simulink model "model_2"  (R2018b)
settings: Solver=FixedStepAuto  StartTime=0.0  StopTime=100  FixedStep=0.0001  MinStep=0.00001  RelTol=1e-5  AbsTol=1e-5
values from neighbouring files (symbols this model uses):
  m = 1    [Drive.m]    (also in on.m)
  N = 1 / T_f    (= 12.8205128205)    [regler.m]
undefined symbols (not defined in the file or in its folder): X, Y, Z
libraries: sm_lib x72, nesl_utility x28, simulink x5, Contact_Forces_Lib x4, simulink_extras x3, vrlib x1
(part 3 of 3)

== system model_2/World/Tracksystem/SensorN6 ==
  Constant : Constant  Value=linePath
  Constant1 : Constant  Value=thickness
  Gain : Gain  Gain=-1
  Gain1 : Gain  Gain=-1
  MATLAB Function2 : MATLAB Function  TreatAsAtomicUnit=on
  PS-Simulink Converter : nesl_utility/PS-Simulink Converter  PhysicalDomain=network_engine_domain  SubClassName=ps_output  LeftPortType=input  RightPortType=output  PseudoPeriodic=off  Frequencies=[]  Unit=1  AffineConversion=off
  PS-Simulink Converter1 : nesl_utility/PS-Simulink Converter  PhysicalDomain=network_engine_domain  SubClassName=ps_output  LeftPortType=input  RightPortType=output  PseudoPeriodic=off  Frequencies=[]  Unit=1  AffineConversion=off
  Scope : Scope  NumInputPorts=2
  Transform Sensor : sm_lib/Frames and Transforms/Transform Sensor  MeasurementFrame=World  SenseAngle=off  SenseAxis=off  SenseAngle1=off  SenseAngle2=off  SenseAngle3=off  SenseQ=off  SenseR=off  SenseOmegaX=off  SenseOmegaY=off  SenseOmegaZ=off  SenseOmega1=off  SenseOmega2=off  SenseOmega3=off  SenseQDot=off  SenseRDot=off  SenseAlphaX=off  SenseAlphaY=off  SenseAlphaZ=off  SenseAlpha1=off  SenseAlpha2=off  SenseAlpha3=off  SenseQDDot=off  SenseRDDot=off  SenseX=on  SenseY=on  SenseZ=off  SenseRad=off  SenseAzim=off  SenseDist=off  SenseInc=off  SenseXDot=off  SenseYDot=off  SenseZDot=off  SenseRadDot=off  SenseAzimDot=off  SenseDistDot=off  SenseIncDot=off  SenseXDDot=off  SenseYDDot=off  SenseZDDot=off  SenseRadDDot=off  SenseAzimDDot=off  SenseDistDDot=off  SenseIncDDot=off
  B : PMIOPort  Side=Left
  Active : Outport
  wires:
  Constant1/1 -> MATLAB Function2/4(thickness)
  Constant/1 -> MATLAB Function2/3(linePath)
  MATLAB Function2/1(b) -> Active/1
  PS-Simulink Converter1/1 -> Gain1/1
  PS-Simulink Converter/1 -> Gain/1
  Gain/1 -> Scope/1, MATLAB Function2/1(x)
  Gain1/1 -> Scope/2, MATLAB Function2/2(y)
  connections:
  Transform Sensor/RConn3 -- PS-Simulink Converter1/LConn1
  Transform Sensor/RConn2 -- PS-Simulink Converter/LConn1
  Transform Sensor/LConn1 -- B/RConn1

== system model_2/World/Tracksystem/SensorN7 ==
  Constant : Constant  Value=linePath
  Constant1 : Constant  Value=thickness
  Gain : Gain  Gain=-1
  Gain1 : Gain  Gain=-1
  MATLAB Function2 : MATLAB Function  TreatAsAtomicUnit=on
  PS-Simulink Converter : nesl_utility/PS-Simulink Converter  PhysicalDomain=network_engine_domain  SubClassName=ps_output  LeftPortType=input  RightPortType=output  PseudoPeriodic=off  Frequencies=[]  Unit=1  AffineConversion=off
  PS-Simulink Converter1 : nesl_utility/PS-Simulink Converter  PhysicalDomain=network_engine_domain  SubClassName=ps_output  LeftPortType=input  RightPortType=output  PseudoPeriodic=off  Frequencies=[]  Unit=1  AffineConversion=off
  Scope : Scope  NumInputPorts=2
  Transform Sensor : sm_lib/Frames and Transforms/Transform Sensor  MeasurementFrame=World  SenseAngle=off  SenseAxis=off  SenseAngle1=off  SenseAngle2=off  SenseAngle3=off  SenseQ=off  SenseR=off  SenseOmegaX=off  SenseOmegaY=off  SenseOmegaZ=off  SenseOmega1=off  SenseOmega2=off  SenseOmega3=off  SenseQDot=off  SenseRDot=off  SenseAlphaX=off  SenseAlphaY=off  SenseAlphaZ=off  SenseAlpha1=off  SenseAlpha2=off  SenseAlpha3=off  SenseQDDot=off  SenseRDDot=off  SenseX=on  SenseY=on  SenseZ=off  SenseRad=off  SenseAzim=off  SenseDist=off  SenseInc=off  SenseXDot=off  SenseYDot=off  SenseZDot=off  SenseRadDot=off  SenseAzimDot=off  SenseDistDot=off  SenseIncDot=off  SenseXDDot=off  SenseYDDot=off  SenseZDDot=off  SenseRadDDot=off  SenseAzimDDot=off  SenseDistDDot=off  SenseIncDDot=off
  B : PMIOPort  Side=Left
  Active : Outport
  wires:
  Constant1/1 -> MATLAB Function2/4(thickness)
  Constant/1 -> MATLAB Function2/3(linePath)
  MATLAB Function2/1(b) -> Active/1
  PS-Simulink Converter1/1 -> Gain1/1
  PS-Simulink Converter/1 -> Gain/1
  Gain/1 -> Scope/1, MATLAB Function2/1(x)
  Gain1/1 -> Scope/2, MATLAB Function2/2(y)
  connections:
  Transform Sensor/RConn3 -- PS-Simulink Converter1/LConn1
  Transform Sensor/RConn2 -- PS-Simulink Converter/LConn1
  Transform Sensor/LConn1 -- B/RConn1

== system model_2/World/Tracksystem/SensorN8 ==
  Constant : Constant  Value=linePath
  Constant1 : Constant  Value=thickness
  Gain : Gain  Gain=-1
  Gain1 : Gain  Gain=-1
  MATLAB Function2 : MATLAB Function  TreatAsAtomicUnit=on
  PS-Simulink Converter : nesl_utility/PS-Simulink Converter  PhysicalDomain=network_engine_domain  SubClassName=ps_output  LeftPortType=input  RightPortType=output  PseudoPeriodic=off  Frequencies=[]  Unit=1  AffineConversion=off
  PS-Simulink Converter1 : nesl_utility/PS-Simulink Converter  PhysicalDomain=network_engine_domain  SubClassName=ps_output  LeftPortType=input  RightPortType=output  PseudoPeriodic=off  Frequencies=[]  Unit=1  AffineConversion=off
  Scope : Scope  NumInputPorts=2
  Transform Sensor : sm_lib/Frames and Transforms/Transform Sensor  MeasurementFrame=World  SenseAngle=off  SenseAxis=off  SenseAngle1=off  SenseAngle2=off  SenseAngle3=off  SenseQ=off  SenseR=off  SenseOmegaX=off  SenseOmegaY=off  SenseOmegaZ=off  SenseOmega1=off  SenseOmega2=off  SenseOmega3=off  SenseQDot=off  SenseRDot=off  SenseAlphaX=off  SenseAlphaY=off  SenseAlphaZ=off  SenseAlpha1=off  SenseAlpha2=off  SenseAlpha3=off  SenseQDDot=off  SenseRDDot=off  SenseX=on  SenseY=on  SenseZ=off  SenseRad=off  SenseAzim=off  SenseDist=off  SenseInc=off  SenseXDot=off  SenseYDot=off  SenseZDot=off  SenseRadDot=off  SenseAzimDot=off  SenseDistDot=off  SenseIncDot=off  SenseXDDot=off  SenseYDDot=off  SenseZDDot=off  SenseRadDDot=off  SenseAzimDDot=off  SenseDistDDot=off  SenseIncDDot=off
  B : PMIOPort  Side=Left
  Active : Outport
  wires:
  Constant1/1 -> MATLAB Function2/4(thickness)
  Constant/1 -> MATLAB Function2/3(linePath)
  MATLAB Function2/1(b) -> Active/1
  PS-Simulink Converter1/1 -> Gain1/1
  PS-Simulink Converter/1 -> Gain/1
  Gain/1 -> Scope/1, MATLAB Function2/1(x)
  Gain1/1 -> Scope/2, MATLAB Function2/2(y)
  connections:
  Transform Sensor/RConn3 -- PS-Simulink Converter1/LConn1
  Transform Sensor/RConn2 -- PS-Simulink Converter/LConn1
  Transform Sensor/LConn1 -- B/RConn1

== system model_2/World/Tracksystem/Subsystem ==
  sensorDownkord : sm_lib/Frames and Transforms/Rigid Transform  TranslationMethod=Cartesian  TranslationStandardOffset=0  TranslationLengthUnit=m  TranslationStandardAxis=-Z  TranslationCartesianOffset=[sensorRadius 0 75/1000]  TranslationROffset=0  TranslationROffsetUnits=m  TranslationZOffset=0  TranslationZOffsetUnits=m  TranslationThetaOffset=0  TranslationThetaOffsetUnits=deg  RotationMethod=None  RotationAngleUnits=deg  RotationStandardAxis=+Z  RotationAngle=45  RotationArbitraryAxis=[0 0 1]  FollAlignAxisA=+X  BaseAlignAxisA=+Y  FollAlignAxisB=+Y  BaseAlignAxisB=+Z  RotationSequenceAxes=FollowerAxes  RotationSequence=XYX  RotationSequenceAngles=[0 0 0]  RotationSequenceAnglesUnits=deg  RotationMatrix=[1 0 0; 0 1 0; 0 0 1]
  sensorDownkord8 : sm_lib/Frames and Transforms/Rigid Transform  TranslationMethod=None  TranslationStandardOffset=0  TranslationLengthUnit=m  TranslationStandardAxis=-Z  TranslationCartesianOffset=[sensorRadius 0 75/1000]  TranslationROffset=0  TranslationROffsetUnits=m  TranslationZOffset=0  TranslationZOffsetUnits=m  TranslationThetaOffset=0  TranslationThetaOffsetUnits=deg  RotationMethod=StandardAxis  RotationAngleUnits=deg  RotationStandardAxis=+Z  RotationAngle=angle  RotationArbitraryAxis=[0 0 1]  FollAlignAxisA=+X  BaseAlignAxisA=+Y  FollAlignAxisB=+Y  BaseAlignAxisB=+Z  RotationSequenceAxes=FollowerAxes  RotationSequence=XYX  RotationSequenceAngles=[0 0 0]  RotationSequenceAnglesUnits=deg  RotationMatrix=[1 0 0; 0 1 0; 0 0 1]
  B : PMIOPort  Side=Left
  F : PMIOPort  Port=2  Side=Right
  connections:
  sensorDownkord8/LConn1 -- B/RConn1
  sensorDownkord/LConn1 -- sensorDownkord8/RConn1
  sensorDownkord/RConn1 -- F/RConn1

== system model_2/World/Tracksystem/Subsystem1 ==
  sensorDownkord : sm_lib/Frames and Transforms/Rigid Transform  TranslationMethod=Cartesian  TranslationStandardOffset=0  TranslationLengthUnit=m  TranslationStandardAxis=-Z  TranslationCartesianOffset=[sensorRadius 0 75/1000]  TranslationROffset=0  TranslationROffsetUnits=m  TranslationZOffset=0  TranslationZOffsetUnits=m  TranslationThetaOffset=0  TranslationThetaOffsetUnits=deg  RotationMethod=None  RotationAngleUnits=deg  RotationStandardAxis=+Z  RotationAngle=45  RotationArbitraryAxis=[0 0 1]  FollAlignAxisA=+X  BaseAlignAxisA=+Y  FollAlignAxisB=+Y  BaseAlignAxisB=+Z  RotationSequenceAxes=FollowerAxes  RotationSequence=XYX  RotationSequenceAngles=[0 0 0]  RotationSequenceAnglesUnits=deg  RotationMatrix=[1 0 0; 0 1 0; 0 0 1]
  sensorDownkord8 : sm_lib/Frames and Transforms/Rigid Transform  TranslationMethod=None  TranslationStandardOffset=0  TranslationLengthUnit=m  TranslationStandardAxis=-Z  TranslationCartesianOffset=[sensorRadius 0 75/1000]  TranslationROffset=0  TranslationROffsetUnits=m  TranslationZOffset=0  TranslationZOffsetUnits=m  TranslationThetaOffset=0  TranslationThetaOffsetUnits=deg  RotationMethod=StandardAxis  RotationAngleUnits=deg  RotationStandardAxis=+Z  RotationAngle=angle  RotationArbitraryAxis=[0 0 1]  FollAlignAxisA=+X  BaseAlignAxisA=+Y  FollAlignAxisB=+Y  BaseAlignAxisB=+Z  RotationSequenceAxes=FollowerAxes  RotationSequence=XYX  RotationSequenceAngles=[0 0 0]  RotationSequenceAnglesUnits=deg  RotationMatrix=[1 0 0; 0 1 0; 0 0 1]
  B : PMIOPort  Side=Left
  F : PMIOPort  Port=2  Side=Right
  connections:
  sensorDownkord8/LConn1 -- B/RConn1
  sensorDownkord/LConn1 -- sensorDownkord8/RConn1
  sensorDownkord/RConn1 -- F/RConn1

== system model_2/World/Tracksystem/Subsystem2 ==
  sensorDownkord : sm_lib/Frames and Transforms/Rigid Transform  TranslationMethod=Cartesian  TranslationStandardOffset=0  TranslationLengthUnit=m  TranslationStandardAxis=-Z  TranslationCartesianOffset=[sensorRadius 0 75/1000]  TranslationROffset=0  TranslationROffsetUnits=m  TranslationZOffset=0  TranslationZOffsetUnits=m  TranslationThetaOffset=0  TranslationThetaOffsetUnits=deg  RotationMethod=None  RotationAngleUnits=deg  RotationStandardAxis=+Z  RotationAngle=45  RotationArbitraryAxis=[0 0 1]  FollAlignAxisA=+X  BaseAlignAxisA=+Y  FollAlignAxisB=+Y  BaseAlignAxisB=+Z  RotationSequenceAxes=FollowerAxes  RotationSequence=XYX  RotationSequenceAngles=[0 0 0]  RotationSequenceAnglesUnits=deg  RotationMatrix=[1 0 0; 0 1 0; 0 0 1]
  sensorDownkord8 : sm_lib/Frames and Transforms/Rigid Transform  TranslationMethod=None  TranslationStandardOffset=0  TranslationLengthUnit=m  TranslationStandardAxis=-Z  TranslationCartesianOffset=[sensorRadius 0 75/1000]  TranslationROffset=0  TranslationROffsetUnits=m  TranslationZOffset=0  TranslationZOffsetUnits=m  TranslationThetaOffset=0  TranslationThetaOffsetUnits=deg  RotationMethod=StandardAxis  RotationAngleUnits=deg  RotationStandardAxis=+Z  RotationAngle=angle  RotationArbitraryAxis=[0 0 1]  FollAlignAxisA=+X  BaseAlignAxisA=+Y  FollAlignAxisB=+Y  BaseAlignAxisB=+Z  RotationSequenceAxes=FollowerAxes  RotationSequence=XYX  RotationSequenceAngles=[0 0 0]  RotationSequenceAnglesUnits=deg  RotationMatrix=[1 0 0; 0 1 0; 0 0 1]
  B : PMIOPort  Side=Left
  F : PMIOPort  Port=2  Side=Right
  connections:
  sensorDownkord8/LConn1 -- B/RConn1
  sensorDownkord/LConn1 -- sensorDownkord8/RConn1
  sensorDownkord/RConn1 -- F/RConn1

== system model_2/World/Tracksystem/Subsystem3 ==
  sensorDownkord : sm_lib/Frames and Transforms/Rigid Transform  TranslationMethod=Cartesian  TranslationStandardOffset=0  TranslationLengthUnit=m  TranslationStandardAxis=-Z  TranslationCartesianOffset=[sensorRadius 0 75/1000]  TranslationROffset=0  TranslationROffsetUnits=m  TranslationZOffset=0  TranslationZOffsetUnits=m  TranslationThetaOffset=0  TranslationThetaOffsetUnits=deg  RotationMethod=None  RotationAngleUnits=deg  RotationStandardAxis=+Z  RotationAngle=45  RotationArbitraryAxis=[0 0 1]  FollAlignAxisA=+X  BaseAlignAxisA=+Y  FollAlignAxisB=+Y  BaseAlignAxisB=+Z  RotationSequenceAxes=FollowerAxes  RotationSequence=XYX  RotationSequenceAngles=[0 0 0]  RotationSequenceAnglesUnits=deg  RotationMatrix=[1 0 0; 0 1 0; 0 0 1]
  sensorDownkord8 : sm_lib/Frames and Transforms/Rigid Transform  TranslationMethod=None  TranslationStandardOffset=0  TranslationLengthUnit=m  TranslationStandardAxis=-Z  TranslationCartesianOffset=[sensorRadius 0 75/1000]  TranslationROffset=0  TranslationROffsetUnits=m  TranslationZOffset=0  TranslationZOffsetUnits=m  TranslationThetaOffset=0  TranslationThetaOffsetUnits=deg  RotationMethod=StandardAxis  RotationAngleUnits=deg  RotationStandardAxis=+Z  RotationAngle=angle  RotationArbitraryAxis=[0 0 1]  FollAlignAxisA=+X  BaseAlignAxisA=+Y  FollAlignAxisB=+Y  BaseAlignAxisB=+Z  RotationSequenceAxes=FollowerAxes  RotationSequence=XYX  RotationSequenceAngles=[0 0 0]  RotationSequenceAnglesUnits=deg  RotationMatrix=[1 0 0; 0 1 0; 0 0 1]
  B : PMIOPort  Side=Left
  F : PMIOPort  Port=2  Side=Right
  connections:
  sensorDownkord8/LConn1 -- B/RConn1
  sensorDownkord/LConn1 -- sensorDownkord8/RConn1
  sensorDownkord/RConn1 -- F/RConn1

== system model_2/World/Tracksystem/Subsystem5 ==
  sensorDownkord : sm_lib/Frames and Transforms/Rigid Transform  TranslationMethod=Cartesian  TranslationStandardOffset=0  TranslationLengthUnit=m  TranslationStandardAxis=-Z  TranslationCartesianOffset=[sensorRadius 0 75/1000]  TranslationROffset=0  TranslationROffsetUnits=m  TranslationZOffset=0  TranslationZOffsetUnits=m  TranslationThetaOffset=0  TranslationThetaOffsetUnits=deg  RotationMethod=None  RotationAngleUnits=deg  RotationStandardAxis=+Z  RotationAngle=45  RotationArbitraryAxis=[0 0 1]  FollAlignAxisA=+X  BaseAlignAxisA=+Y  FollAlignAxisB=+Y  BaseAlignAxisB=+Z  RotationSequenceAxes=FollowerAxes  RotationSequence=XYX  RotationSequenceAngles=[0 0 0]  RotationSequenceAnglesUnits=deg  RotationMatrix=[1 0 0; 0 1 0; 0 0 1]
  sensorDownkord8 : sm_lib/Frames and Transforms/Rigid Transform  TranslationMethod=None  TranslationStandardOffset=0  TranslationLengthUnit=m  TranslationStandardAxis=-Z  TranslationCartesianOffset=[sensorRadius 0 75/1000]  TranslationROffset=0  TranslationROffsetUnits=m  TranslationZOffset=0  TranslationZOffsetUnits=m  TranslationThetaOffset=0  TranslationThetaOffsetUnits=deg  RotationMethod=StandardAxis  RotationAngleUnits=deg  RotationStandardAxis=+Z  RotationAngle=angle  RotationArbitraryAxis=[0 0 1]  FollAlignAxisA=+X  BaseAlignAxisA=+Y  FollAlignAxisB=+Y  BaseAlignAxisB=+Z  RotationSequenceAxes=FollowerAxes  RotationSequence=XYX  RotationSequenceAngles=[0 0 0]  RotationSequenceAnglesUnits=deg  RotationMatrix=[1 0 0; 0 1 0; 0 0 1]
  B : PMIOPort  Side=Left
  F : PMIOPort  Port=2  Side=Right
  connections:
  sensorDownkord8/LConn1 -- B/RConn1
  sensorDownkord/LConn1 -- sensorDownkord8/RConn1
  sensorDownkord/RConn1 -- F/RConn1

== system model_2/World/Tracksystem/Subsystem6 ==
  sensorDownkord : sm_lib/Frames and Transforms/Rigid Transform  TranslationMethod=Cartesian  TranslationStandardOffset=0  TranslationLengthUnit=m  TranslationStandardAxis=-Z  TranslationCartesianOffset=[sensorRadius 0 75/1000]  TranslationROffset=0  TranslationROffsetUnits=m  TranslationZOffset=0  TranslationZOffsetUnits=m  TranslationThetaOffset=0  TranslationThetaOffsetUnits=deg  RotationMethod=None  RotationAngleUnits=deg  RotationStandardAxis=+Z  RotationAngle=45  RotationArbitraryAxis=[0 0 1]  FollAlignAxisA=+X  BaseAlignAxisA=+Y  FollAlignAxisB=+Y  BaseAlignAxisB=+Z  RotationSequenceAxes=FollowerAxes  RotationSequence=XYX  RotationSequenceAngles=[0 0 0]  RotationSequenceAnglesUnits=deg  RotationMatrix=[1 0 0; 0 1 0; 0 0 1]
  sensorDownkord8 : sm_lib/Frames and Transforms/Rigid Transform  TranslationMethod=None  TranslationStandardOffset=0  TranslationLengthUnit=m  TranslationStandardAxis=-Z  TranslationCartesianOffset=[sensorRadius 0 75/1000]  TranslationROffset=0  TranslationROffsetUnits=m  TranslationZOffset=0  TranslationZOffsetUnits=m  TranslationThetaOffset=0  TranslationThetaOffsetUnits=deg  RotationMethod=StandardAxis  RotationAngleUnits=deg  RotationStandardAxis=+Z  RotationAngle=angle  RotationArbitraryAxis=[0 0 1]  FollAlignAxisA=+X  BaseAlignAxisA=+Y  FollAlignAxisB=+Y  BaseAlignAxisB=+Z  RotationSequenceAxes=FollowerAxes  RotationSequence=XYX  RotationSequenceAngles=[0 0 0]  RotationSequenceAnglesUnits=deg  RotationMatrix=[1 0 0; 0 1 0; 0 0 1]
  B : PMIOPort  Side=Left
  F : PMIOPort  Port=2  Side=Right
  connections:
  sensorDownkord8/LConn1 -- B/RConn1
  sensorDownkord/LConn1 -- sensorDownkord8/RConn1
  sensorDownkord/RConn1 -- F/RConn1

== system model_2/World/Tracksystem/Subsystem7 ==
  sensorDownkord : sm_lib/Frames and Transforms/Rigid Transform  TranslationMethod=Cartesian  TranslationStandardOffset=0  TranslationLengthUnit=m  TranslationStandardAxis=-Z  TranslationCartesianOffset=[sensorRadius 0 75/1000]  TranslationROffset=0  TranslationROffsetUnits=m  TranslationZOffset=0  TranslationZOffsetUnits=m  TranslationThetaOffset=0  TranslationThetaOffsetUnits=deg  RotationMethod=None  RotationAngleUnits=deg  RotationStandardAxis=+Z  RotationAngle=45  RotationArbitraryAxis=[0 0 1]  FollAlignAxisA=+X  BaseAlignAxisA=+Y  FollAlignAxisB=+Y  BaseAlignAxisB=+Z  RotationSequenceAxes=FollowerAxes  RotationSequence=XYX  RotationSequenceAngles=[0 0 0]  RotationSequenceAnglesUnits=deg  RotationMatrix=[1 0 0; 0 1 0; 0 0 1]
  sensorDownkord8 : sm_lib/Frames and Transforms/Rigid Transform  TranslationMethod=None  TranslationStandardOffset=0  TranslationLengthUnit=m  TranslationStandardAxis=-Z  TranslationCartesianOffset=[sensorRadius 0 75/1000]  TranslationROffset=0  TranslationROffsetUnits=m  TranslationZOffset=0  TranslationZOffsetUnits=m  TranslationThetaOffset=0  TranslationThetaOffsetUnits=deg  RotationMethod=StandardAxis  RotationAngleUnits=deg  RotationStandardAxis=+Z  RotationAngle=angle  RotationArbitraryAxis=[0 0 1]  FollAlignAxisA=+X  BaseAlignAxisA=+Y  FollAlignAxisB=+Y  BaseAlignAxisB=+Z  RotationSequenceAxes=FollowerAxes  RotationSequence=XYX  RotationSequenceAngles=[0 0 0]  RotationSequenceAnglesUnits=deg  RotationMatrix=[1 0 0; 0 1 0; 0 0 1]
  B : PMIOPort  Side=Left
  F : PMIOPort  Port=2  Side=Right
  connections:
  sensorDownkord8/LConn1 -- B/RConn1
  sensorDownkord/LConn1 -- sensorDownkord8/RConn1
  sensorDownkord/RConn1 -- F/RConn1

== system model_2/World/Tracksystem/Subsystem8 ==
  sensorDownkord : sm_lib/Frames and Transforms/Rigid Transform  TranslationMethod=Cartesian  TranslationStandardOffset=0  TranslationLengthUnit=m  TranslationStandardAxis=-Z  TranslationCartesianOffset=[sensorRadius 0 75/1000]  TranslationROffset=0  TranslationROffsetUnits=m  TranslationZOffset=0  TranslationZOffsetUnits=m  TranslationThetaOffset=0  TranslationThetaOffsetUnits=deg  RotationMethod=None  RotationAngleUnits=deg  RotationStandardAxis=+Z  RotationAngle=45  RotationArbitraryAxis=[0 0 1]  FollAlignAxisA=+X  BaseAlignAxisA=+Y  FollAlignAxisB=+Y  BaseAlignAxisB=+Z  RotationSequenceAxes=FollowerAxes  RotationSequence=XYX  RotationSequenceAngles=[0 0 0]  RotationSequenceAnglesUnits=deg  RotationMatrix=[1 0 0; 0 1 0; 0 0 1]
  sensorDownkord8 : sm_lib/Frames and Transforms/Rigid Transform  TranslationMethod=None  TranslationStandardOffset=0  TranslationLengthUnit=m  TranslationStandardAxis=-Z  TranslationCartesianOffset=[sensorRadius 0 75/1000]  TranslationROffset=0  TranslationROffsetUnits=m  TranslationZOffset=0  TranslationZOffsetUnits=m  TranslationThetaOffset=0  TranslationThetaOffsetUnits=deg  RotationMethod=StandardAxis  RotationAngleUnits=deg  RotationStandardAxis=+Z  RotationAngle=angle  RotationArbitraryAxis=[0 0 1]  FollAlignAxisA=+X  BaseAlignAxisA=+Y  FollAlignAxisB=+Y  BaseAlignAxisB=+Z  RotationSequenceAxes=FollowerAxes  RotationSequence=XYX  RotationSequenceAngles=[0 0 0]  RotationSequenceAnglesUnits=deg  RotationMatrix=[1 0 0; 0 1 0; 0 0 1]
  B : PMIOPort  Side=Left
  F : PMIOPort  Port=2  Side=Right
  connections:
  sensorDownkord8/LConn1 -- B/RConn1
  sensorDownkord/LConn1 -- sensorDownkord8/RConn1
  sensorDownkord/RConn1 -- F/RConn1

== matlab function model_2/World/Car/Wheel Model 1/MATLAB Function ==
  data: vector input; y output; saturate input
function y = fcn(vector, saturate)
	y = vector/norm(vector) * max(-saturate, min(saturate, norm(vector)));

== matlab function model_2/World/Car/Wheel Model 2/MATLAB Function ==
  data: vector input; y output; saturate input
function y = fcn(vector, saturate)
	y = vector/norm(vector) * max(-saturate, min(saturate, norm(vector)));

== matlab function model_2/World/Car/Wheel Model 3/MATLAB Function ==
  data: vector input; y output; saturate input
function y = fcn(vector, saturate)
	y = vector/norm(vector) * max(-saturate, min(saturate, norm(vector)));

== matlab function model_2/World/Car/Wheel Model 4/MATLAB Function ==
  data: vector input; y output; saturate input
function y = fcn(vector, saturate)
	y = vector/norm(vector) * max(-saturate, min(saturate, norm(vector)));

== matlab function model_2/World/Heading Regulator/MATLAB Function ==
  data: u input; y output
function y = fcn(u)
	if (u >= pi)
		u = u-2*pi;
	elseif (u <= -pi)
		u = u+2*pi;
	end
y = u;

== matlab function model_2/World/MATLAB Function1 ==
  data: t input; y output
function y = fcn(t)
	u = [0.6; 0.3];
y = u;

== matlab function model_2/World/MATLAB Function2 ==
  data: t input; y output
function y = fcn(t)
	u = 0;
y = u;

== matlab function model_2/World/Tracksystem/SensorN1/MATLAB Function2 ==
  data: x input; b output; y input; linePath input; thickness input
function b = fcn(x, y, linePath, thickness)
	b = 0;

	for i = 1 : length(linePath)-1
		p0 = [x y];

		p1 = linePath(i,:);
		p2 = linePath(i+1,:);

		p = p2 - p1;

		angle = -atan2(p(2), p(1));

		A = [
			cos(angle) -sin(angle)
			sin(angle)	cos(angle)
		];

		p0 = A*transpose(p0);
		p1 = A*transpose(p1);
		p2 = A*transpose(p2);

		if or(and(p0(1) >= p1(1), p0(1) <= p2(1)), and(p0(1) >= p2(1), p0(1) <= p1(1)))
			% IT IS INBETWEEN! COMPARE Y COORDS
			if abs(p0(2)-p1(2)) <= thickness
				% WE ARE POSITIVE
				b = 1;
				break;
			end
		elseif min(norm(p1-p0), norm(p2-p0)) <= thickness
			b = 1;
			break;
		end
		
	end

== matlab function model_2/World/Tracksystem/SensorN2/MATLAB Function2 ==
  data: x input; b output; y input; linePath input; thickness input
function b = fcn(x, y, linePath, thickness)
	b = 0;

	for i = 1 : length(linePath)-1
		p0 = [x y];

		p1 = linePath(i,:);
		p2 = linePath(i+1,:);

		p = p2 - p1;

		angle = -atan2(p(2), p(1));

		A = [
			cos(angle) -sin(angle)
			sin(angle)	cos(angle)
		];

		p0 = A*transpose(p0);
		p1 = A*transpose(p1);
		p2 = A*transpose(p2);

		if or(and(p0(1) >= p1(1), p0(1) <= p2(1)), and(p0(1) >= p2(1), p0(1) <= p1(1)))
			% IT IS INBETWEEN! COMPARE Y COORDS
			if abs(p0(2)-p1(2)) <= thickness
				% WE ARE POSITIVE
				b = 1;
				break;
			end
		elseif min(norm(p1-p0), norm(p2-p0)) <= thickness
			b = 1;
			break;
		end
		
	end

== matlab function model_2/World/Tracksystem/SensorN3/MATLAB Function2 ==
  data: x input; b output; y input; linePath input; thickness input
function b = fcn(x, y, linePath, thickness)
	b = 0;

	for i = 1 : length(linePath)-1
		p0 = [x y];

		p1 = linePath(i,:);
		p2 = linePath(i+1,:);

		p = p2 - p1;

		angle = -atan2(p(2), p(1));

		A = [
			cos(angle) -sin(angle)
			sin(angle)	cos(angle)
		];

		p0 = A*transpose(p0);
		p1 = A*transpose(p1);
		p2 = A*transpose(p2);

		if or(and(p0(1) >= p1(1), p0(1) <= p2(1)), and(p0(1) >= p2(1), p0(1) <= p1(1)))
			% IT IS INBETWEEN! COMPARE Y COORDS
			if abs(p0(2)-p1(2)) <= thickness
				% WE ARE POSITIVE
				b = 1;
				break;
			end
		elseif min(norm(p1-p0), norm(p2-p0)) <= thickness
			b = 1;
			break;
		end
		
	end

== matlab function model_2/World/Tracksystem/SensorN4/MATLAB Function2 ==
  data: x input; b output; y input; linePath input; thickness input
function b = fcn(x, y, linePath, thickness)
	b = 0;

	for i = 1 : length(linePath)-1
		p0 = [x y];

		p1 = linePath(i,:);
		p2 = linePath(i+1,:);

		p = p2 - p1;

		angle = -atan2(p(2), p(1));

		A = [
			cos(angle) -sin(angle)
			sin(angle)	cos(angle)
		];

		p0 = A*transpose(p0);
		p1 = A*transpose(p1);
		p2 = A*transpose(p2);

		if or(and(p0(1) >= p1(1), p0(1) <= p2(1)), and(p0(1) >= p2(1), p0(1) <= p1(1)))
			% IT IS INBETWEEN! COMPARE Y COORDS
			if abs(p0(2)-p1(2)) <= thickness
				% WE ARE POSITIVE
				b = 1;
				break;
			end
		elseif min(norm(p1-p0), norm(p2-p0)) <= thickness
			b = 1;
			break;
		end
		
	end

== matlab function model_2/World/Tracksystem/SensorN7/MATLAB Function2 ==
  data: x input; b output; y input; linePath input; thickness input
function b = fcn(x, y, linePath, thickness)
	b = 0;

	for i = 1 : length(linePath)-1
		p0 = [x y];

		p1 = linePath(i,:);
		p2 = linePath(i+1,:);

		p = p2 - p1;

		angle = -atan2(p(2), p(1));

		A = [
			cos(angle) -sin(angle)
			sin(angle)	cos(angle)
		];

		p0 = A*transpose(p0);
		p1 = A*transpose(p1);
		p2 = A*transpose(p2);

		if or(and(p0(1) >= p1(1), p0(1) <= p2(1)), and(p0(1) >= p2(1), p0(1) <= p1(1)))
			% IT IS INBETWEEN! COMPARE Y COORDS
			if abs(p0(2)-p1(2)) <= thickness
				% WE ARE POSITIVE
				b = 1;
				break;
			end
		elseif min(norm(p1-p0), norm(p2-p0)) <= thickness
			b = 1;
			break;
		end
		
	end

== matlab function model_2/World/Tracksystem/SensorN5/MATLAB Function2 ==
  data: x input; b output; y input; linePath input; thickness input
function b = fcn(x, y, linePath, thickness)
	b = 0;

	for i = 1 : length(linePath)-1
		p0 = [x y];

		p1 = linePath(i,:);
		p2 = linePath(i+1,:);

		p = p2 - p1;

		angle = -atan2(p(2), p(1));

		A = [
			cos(angle) -sin(angle)
			sin(angle)	cos(angle)
		];

		p0 = A*transpose(p0);
		p1 = A*transpose(p1);
		p2 = A*transpose(p2);

		if or(and(p0(1) >= p1(1), p0(1) <= p2(1)), and(p0(1) >= p2(1), p0(1) <= p1(1)))
			% IT IS INBETWEEN! COMPARE Y COORDS
			if abs(p0(2)-p1(2)) <= thickness
				% WE ARE POSITIVE
				b = 1;
				break;
			end
		elseif min(norm(p1-p0), norm(p2-p0)) <= thickness
			b = 1;
			break;
		end
		
	end

== matlab function model_2/World/Tracksystem/SensorN8/MATLAB Function2 ==
  data: x input; b output; y input; linePath input; thickness input
function b = fcn(x, y, linePath, thickness)
	b = 0;

	for i = 1 : length(linePath)-1
		p0 = [x y];

		p1 = linePath(i,:);
		p2 = linePath(i+1,:);

		p = p2 - p1;

		angle = -atan2(p(2), p(1));

		A = [
			cos(angle) -sin(angle)
			sin(angle)	cos(angle)
		];

		p0 = A*transpose(p0);
		p1 = A*transpose(p1);
		p2 = A*transpose(p2);

		if or(and(p0(1) >= p1(1), p0(1) <= p2(1)), and(p0(1) >= p2(1), p0(1) <= p1(1)))
			% IT IS INBETWEEN! COMPARE Y COORDS
			if abs(p0(2)-p1(2)) <= thickness
				% WE ARE POSITIVE
				b = 1;
				break;
			end
		elseif min(norm(p1-p0), norm(p2-p0)) <= thickness
			b = 1;
			break;
		end
		
	end

== matlab function model_2/World/MATLAB Function3 ==
  data: t input; y output
function y = fcn(t)
	u = 0;
	
	if (t > 5)
		u = -0.15;
	end
y = u;

== matlab function model_2/World/Tracksystem/SensorN6/MATLAB Function2 ==
  data: x input; b output; y input; linePath input; thickness input
function b = fcn(x, y, linePath, thickness)
	b = 0;

	for i = 1 : length(linePath)-1
		p0 = [x y];

		p1 = linePath(i,:);
		p2 = linePath(i+1,:);

		p = p2 - p1;

		angle = -atan2(p(2), p(1));

		A = [
			cos(angle) -sin(angle)
			sin(angle)	cos(angle)
		];

		p0 = A*transpose(p0);
		p1 = A*transpose(p1);
		p2 = A*transpose(p2);

		if or(and(p0(1) >= p1(1), p0(1) <= p2(1)), and(p0(1) >= p2(1), p0(1) <= p1(1)))
			% IT IS INBETWEEN! COMPARE Y COORDS
			if abs(p0(2)-p1(2)) <= thickness
				% WE ARE POSITIVE
				b = 1;
				break;
			end
		elseif min(norm(p1-p0), norm(p2-p0)) <= thickness
			b = 1;
			break;
		end
		
	end

== matlab function model_2/World/Axis Rotater/MATLAB Function ==
  data: u input; y output
function y = fcn(u)
	cosu = cos(u);
	sinu = sin(u);
	
	y = [
		cosu -sinu
		sinu  cosu
	];

== matlab function model_2/World/MATLAB Function5 ==
  settings: updateMethod=DISCRETE  sampleTime=0.0001
  data: t input; activeSens input; activeSensOld input; driveDir output; driveSensOld input; driveSens output; lastAddedDriveSensOld input; lastAddedDriveSens output; lastDrivenInPairOld input; lastDrivenInPair output
function [driveDir,driveSens,lastAddedDriveSens,lastDrivenInPair]= fcn(t, activeSens,activeSensOld,driveSensOld,lastAddedDriveSensOld,lastDrivenInPairOld)
%, drivesens1,drivesens2,drivesens3,drivesens4,drivesens5,drivesens6,drivesens7,drivesens8,lastDrivenInPair, lastDrivenInPair1,lastDrivenInPair2,lastDrivenInPair3,lastDrivenInPair4
timeInterval = 0.005;
lastDrivenInPair = lastDrivenInPairOld;
driveDir = [0;0;0;0];
driveSens = driveSensOld;
lastAddedDriveSens = lastAddedDriveSensOld; %De två senaste tillagda drivande sensorerna + tiden då de lades till


for i = 1:1:8
    
    complement = Complement(i,driveSens);
    
    if(activeSensOld(i) == 0 && activeSens(i) == 1 && on(i,driveSens) == 1)
        
        [driveSens,lastAddedDriveSens,lastDrivenInPair] = Drive(i,driveSens,t,lastAddedDriveSens,lastDrivenInPair);
        
        
    elseif(activeSensOld(i) == 0 && activeSens(i) == 1 && complement == 0 && driveSens(lastAddedDriveSens(1)) == 1 && ((abs(i - lastAddedDriveSens(1)) < 2) || (i == 8 && lastAddedDriveSens(1) == 1) || (i == 1 && lastAddedDriveSens(1) == 8)))
        [driveSens,lastAddedDriveSens,lastDrivenInPair] = Drive(i,driveSens,t,lastAddedDriveSens,lastDrivenInPair);
        
    elseif(complement == 0 && (activeSensOld(i) == 0 && activeSens(i) == 1 && driveSens(lastAddedDriveSens(3)) == 1 && abs(lastAddedDriveSens(2)-lastAddedDriveSens(4)) < 0.25 &&((abs(i - lastAddedDriveSens(3)) < 2) || (i == 8 && lastAddedDriveSens(3) == 1) || (i == 1 && lastAddedDriveSens(3) == 8))))
        [driveSens,lastAddedDriveSens,lastDrivenInPair] = Drive(i,driveSens,t,lastAddedDriveSens,lastDrivenInPair);
        
    elseif(activeSens(i) == 0)
        driveSens(i) = 0;
    else
        
    end
end


%Nedanstående loop är för låg hastighet i skarpa kurvor
for i = 1:1:4
    if(activeSensOld(i) == 0 && activeSens(i) == 1 && lastAddedDriveSens(1) == i + 4 && abs(lastAddedDriveSens(2) - t) < timeInterval && lastDrivenInPair(i+4) == 0)
        [driveSens,lastAddedDriveSens,lastDrivenInPair] = Drive(i,driveSens,t,lastAddedDriveSens,lastDrivenInPair);
        
        if(i == 1)
            if(activeSens(2) == 1)
                [driveSens,lastAddedDriveSens,lastDrivenInPair] = Drive(2,driveSens,t,lastAddedDriveSens,lastDrivenInPair);
            end
            if(activeSens(8) == 1)
                [driveSens,lastAddedDriveSens,lastDrivenInPair] = Drive(8,driveSens,t,lastAddedDriveSens,lastDrivenInPair);
            end
        elseif(i == 2)
            if(activeSens(3) == 1)
                [driveSens,lastAddedDriveSens,lastDrivenInPair] = Drive(3,driveSens,t,lastAddedDriveSens,lastDrivenInPair);
            end
            if(activeSens(1) == 1)
                [driveSens,lastAddedDriveSens,lastDrivenInPair] = Drive(1,driveSens,t,lastAddedDriveSens,lastDrivenInPair);
            end
        elseif(i == 3)
            if(activeSens(4) == 1)
                [driveSens,lastAddedDriveSens,lastDrivenInPair] = Drive(4,driveSens,t,lastAddedDriveSens,lastDrivenInPair);
                
            end
            if(activeSens(2) == 1)
                [driveSens,lastAddedDriveSens,lastDrivenInPair] = Drive(2,driveSens,t,lastAddedDriveSens,lastDrivenInPair);
                
            end
        elseif(i == 4)
            if(activeSens(5) == 1)
                [driveSens,lastAddedDriveSens,lastDrivenInPair] = Drive(5,driveSens,t,lastAddedDriveSens,lastDrivenInPair);
                
            end
            if(activeSens(3) == 1)
                [driveSens,lastAddedDriveSens,lastDrivenInPair] = Drive(3,driveSens,t,lastAddedDriveSens,lastDrivenInPair);
                
            end
        end
        
        
    end
    
    if(activeSensOld(i + 4) == 0 && activeSens(i + 4) == 1 && lastAddedDriveSens(1) == i  && abs(lastAddedDriveSens(2) - t) < timeInterval && lastDrivenInPair(i+4) == 1)
        [driveSens,lastAddedDriveSens,lastDrivenInPair] = Drive(i+4,driveSens,t,lastAddedDriveSens,lastDrivenInPair);
        
        
        if(i == 1)
            if(activeSens(6) == 1)
                [driveSens,lastAddedDriveSens,lastDrivenInPair] = Drive(6,driveSens,t,lastAddedDriveSens,lastDrivenInPair);
            end
            if(activeSens(4) == 1)
                [driveSens,lastAddedDriveSens,lastDrivenInPair] = Drive(4,driveSens,t,lastAddedDriveSens,lastDrivenInPair);
            end
        end
        
        if(i == 2)
            if(activeSens(7) == 1)
                [driveSens,lastAddedDriveSens,lastDrivenInPair] = Drive(7,driveSens,t,lastAddedDriveSens,lastDrivenInPair);
            end
            if(activeSens(5) == 1)
                [driveSens,lastAddedDriveSens,lastDrivenInPair] = Drive(5,driveSens,t,lastAddedDriveSens,lastDrivenInPair);
            end
        end
        
        if(i == 3)
            if(activeSens(8) == 1)
                [driveSens,lastAddedDriveSens,lastDrivenInPair] = Drive(8,driveSens,t,lastAddedDriveSens,lastDrivenInPair);
            end
            if(activeSens(6) == 1)
                [driveSens,lastAddedDriveSens,lastDrivenInPair] = Drive(6,driveSens,t,lastAddedDriveSens,lastDrivenInPair);
            end
        end
        
        if(i == 4)
            if(activeSens(1) == 1)
                [driveSens,lastAddedDriveSens,lastDrivenInPair] = Drive(1,driveSens,t,lastAddedDriveSens,lastDrivenInPair);
            end
            if(activeSens(7) == 1)
                [driveSens,lastAddedDriveSens,lastDrivenInPair] = Drive(7,driveSens,t,lastAddedDriveSens,lastDrivenInPair);
            end
        end
        
        
    end
    
end




for i = 1:1:4
    if(driveSens(i) == 1)
        driveDir(i) = 1;
    elseif(driveSens(i+4) == 1)
        driveDir(i) = -1;
    else
        driveDir(i) = 0.001;
    end
end
% lastDrivenInPair1 = lastDrivenInPair(1);
% lastDrivenInPair2 =lastDrivenInPair(2);
% lastDrivenInPair3 = lastDrivenInPair(3);
% lastDrivenInPair4 = lastDrivenInPair(4);
%
% drivesens1 = driveSens(1);
% drivesens2 = driveSens(2);
% drivesens3 = driveSens(3);
% drivesens4 = driveSens(4);
% drivesens5 = driveSens(5);
% drivesens6 = driveSens(6);
% drivesens7 = driveSens(7);
% drivesens8 = driveSens(8);

== matlab function model_2/World/MATLAB Function4 ==
  data: vector input; y output; saturate input
function y = fcn(vector, saturate)
	y = vector/norm(vector) * max(-saturate, min(saturate, norm(vector)));

== matlab function model_2/World/MATLAB Function6 ==
  data: t input; y output
function y = fcn(t)
	u = 0;
	
	if (t > 5)
		u = -1;
	end
y = u;
